simulink model "task1"  (R2022b)
settings: Solver=VariableStepAuto  StartTime=0.0  StopTime=20.0  RelTol=1e-7  AbsTol=1e-7
settings Model: Creator=Иван Бакланов  LastModifiedBy=Иван Бакланов

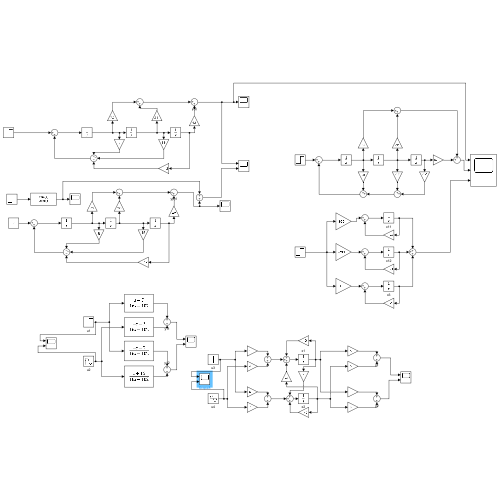
[thumbnail: Simulink's stored preview of the top-level diagram]
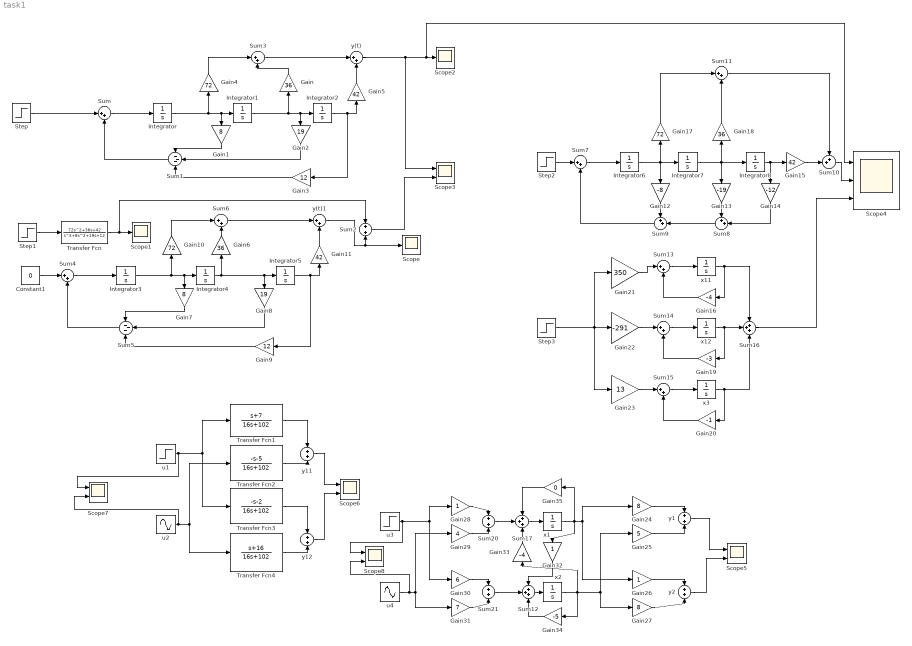
== system task1 ==
  Constant1 : Constant  Value=0
  Gain : Gain  Gain=36
  Gain{1,7,24,27} (4 alike) : Gain  Gain=8
  Gain10 : Gain  Gain=72
  Gain11 : Gain  Gain=42
  Gain12 : Gain  Gain=-8
  Gain13 : Gain  Gain=-19
  Gain14 : Gain  Gain=-12
  Gain15 : Gain  Gain=42
  Gain16 : Gain  Gain=-4
  Gain17 : Gain  Gain=72
  Gain18 : Gain  Gain=36
  Gain19 : Gain  Gain=-3
  Gain2 : Gain  Gain=19
  Gain20 : Gain  Gain=-1
  Gain21 : Gain  Gain=350
  Gain22 : Gain  Gain=-291
  Gain23 : Gain  Gain=13
  Gain25 : Gain  Gain=5
  Gain26 : Gain
  Gain28 : Gain
  Gain29 : Gain  Gain=4
  Gain3 : Gain  Gain=12
  Gain30 : Gain  Gain=6
  Gain31 : Gain  Gain=7
  Gain32 : Gain
  Gain33 : Gain  Gain=-4
  Gain34 : Gain  Gain=-5
  Gain35 : Gain  Gain=0
  Gain4 : Gain  Gain=72
  Gain5 : Gain  Gain=42
  Gain6 : Gain  Gain=36
  Gain8 : Gain  Gain=19
  Gain9 : Gain  Gain=12
  Integrator : Integrator  InitialCondition=0.00743
  Integrator1 : Integrator  InitialCondition=-0.02440
  Integrator2 : Integrator  InitialCondition=0.03199
  Integrator3 : Integrator  InitialCondition=0.00743
  Integrator4 : Integrator  InitialCondition=-0.02440
  Integrator5 : Integrator  InitialCondition=0.03199
  Integrator6 : Integrator  InitialCondition=0.00743
  Integrator7 : Integrator  InitialCondition=-0.02440
  Integrator8 : Integrator  InitialCondition=0.03199
  Scope : Scope
  Scope1 : Scope
  Scope2 : Scope
  Scope{3,5..8} (5 alike) : Scope  NumInputPorts=2
  Scope4 : Scope  NumInputPorts=3
  Step{,1..3} (4 alike) : Step  Time=0  SampleTime=0
  Sum{,3..4,6..7,11,13..15} (9 alike) : Sum  Inputs=|++
  Sum1 : Sum  Inputs=---
  Sum10 : Sum  Inputs=++|
  Sum12 : Sum  Inputs=+++
  Sum16 : Sum  Inputs=+++
  Sum17 : Sum  Inputs=+++
  Sum2 : Sum
  Sum20 : Sum
  Sum21 : Sum
  Sum5 : Sum  Inputs=---
  Sum8 : Sum  Inputs=++|
  Sum9 : Sum  Inputs=++|
  Transfer Fcn : TransferFcn  Numerator=[72 36 42]  Denominator=[1 8 19 12]
  Transfer Fcn1 : TransferFcn  Numerator=[1 7]  Denominator=[16 102]
  Transfer Fcn2 : TransferFcn  Numerator=[-1 -5]  Denominator=[16 102]
  Transfer Fcn3 : TransferFcn  Numerator=[-1 -2]  Denominator=[16 102]
  Transfer Fcn4 : TransferFcn  Numerator=[1 16]  Denominator=[16 102]
  u1 : Step  Time=0  SampleTime=0
  u2 : Sin  SampleTime=0
  u3 : Step  Time=0  SampleTime=0
  u4 : Sin  SampleTime=0
  x1 : Integrator
  x11 : Integrator  InitialCondition=2.0333
  x12 : Integrator  InitialCondition=-3.9
  x2 : Integrator
  x3 : Integrator  InitialCondition=2.86667
  y(t) : Sum  Inputs=|++
  y(t)1 : Sum  Inputs=|++
  y{1..2,11..12} (4 alike) : Sum
  wires:
  Step1/1 -> Transfer Fcn/1
  Transfer Fcn/1 -> Sum2/1, Scope1/1
  Sum/1 -> Integrator/1
  Sum1/1 -> Sum/2
  Sum3/1 -> y(t)/1
  Integrator/1 -> Gain4/1, Gain1/1, Integrator1/1
  Integrator1/1 -> Gain2/1, Integrator2/1, Gain/1
  Integrator2/1 -> Gain3/1, Gain5/1
  Gain4/1 -> Sum3/1
  Gain/1 -> Sum3/2
  Gain5/1 -> y(t)/2
  Gain1/1 -> Sum1/1
  Gain2/1 -> Sum1/2
  Gain3/1 -> Sum1/3
  Integrator5/1 -> Gain9/1, Gain11/1
  Integrator3/1 -> Gain10/1, Gain7/1, Integrator4/1
  Gain11/1 -> y(t)1/2
  Sum5/1 -> Sum4/2
  Gain10/1 -> Sum6/1
  Gain7/1 -> Sum5/1
  Integrator4/1 -> Gain8/1, Integrator5/1, Gain6/1
  Gain8/1 -> Sum5/2
  Sum4/1 -> Integrator3/1
  Gain6/1 -> Sum6/2
  Sum6/1 -> y(t)1/1
  Gain9/1 -> Sum5/3
  Constant1/1 -> Sum4/1
  Sum2/1 -> Scope3/2
  y(t)/1 -> Scope4/1, Scope2/1, Scope3/1
  Step/1 -> Sum/1
  y(t)1/1 -> Scope/1, Sum2/2
  Sum7/1 -> Integrator6/1
  Integrator6/1 -> Gain17/1, Gain12/1, Integrator7/1
  Integrator7/1 -> Gain13/1, Gain18/1, Integrator8/1
  Integrator8/1 -> Gain15/1, Gain14/1
  Gain12/1 -> Sum9/1
  Gain15/1 -> Sum10/2
  Gain18/1 -> Sum11/2
  Step2/1 -> Sum7/1
  Sum9/1 -> Sum7/2
  Sum11/1 -> Sum10/1
  Gain17/1 -> Sum11/1
  Gain13/1 -> Sum8/1
  Sum8/1 -> Sum9/2
  Gain14/1 -> Sum8/2
  Sum13/1 -> x11/1
  x11/1 -> Sum16/1, Gain16/1
  Gain16/1 -> Sum13/2
  Sum14/1 -> x12/1
  Gain19/1 -> Sum14/2
  x12/1 -> Sum16/2, Gain19/1
  Sum15/1 -> x3/1
  Gain20/1 -> Sum15/2
  x3/1 -> Sum16/3, Gain20/1
  Step3/1 -> Gain23/1, Gain22/1, Gain21/1
  Gain22/1 -> Sum14/1
  Gain21/1 -> Sum13/1
  Gain23/1 -> Sum15/1
  Sum10/1 -> Scope4/2
  Sum16/1 -> Scope4/3
  u1/1 -> Scope7/1, Transfer Fcn3/1, Transfer Fcn1/1
  u2/1 -> Scope7/2, Transfer Fcn4/1, Transfer Fcn2/1
  Transfer Fcn1/1 -> y11/1
  Transfer Fcn2/1 -> y11/2
  Transfer Fcn3/1 -> y12/1
  Transfer Fcn4/1 -> y12/2
  y11/1 -> Scope6/1
  y12/1 -> Scope6/2
  Sum12/1 -> x2/1
  Sum17/1 -> x1/1
  x2/1 -> Gain34/1, Gain27/1, Gain25/1, Gain33/1
  x1/1 -> Gain24/1, Gain26/1, Gain35/1, Gain32/1
  Gain27/1 -> y2/2
  y2/1 -> Scope5/2
  Gain26/1 -> y2/1
  Gain25/1 -> y1/2
  Gain24/1 -> y1/1
  y1/1 -> Scope5/1
  u3/1 -> Scope8/1, Gain28/1, Gain30/1
  u4/1 -> Scope8/2, Gain29/1, Gain31/1
  Gain30/1 -> Sum21/1
  Gain31/1 -> Sum21/2
  Gain29/1 -> Sum20/2
  Gain28/1 -> Sum20/1
  Sum20/1 -> Sum17/2
  Sum21/1 -> Sum12/2
  Gain32/1 -> Sum12/1
  Gain33/1 -> Sum17/3
  Gain34/1 -> Sum12/3
  Gain35/1 -> Sum17/1
